simulink model "Hybrid_P2_Parallel_ETE"  (R2017b)
settings: Solver=FixedStepAuto  StartTime=0.0  StopTime=length(Speed)  FixedStep=0.01  MaxStep=0.01  RelTol=1e-3  EnableMultiTasking=on
PostLoadFcn:
  | , if any(exist('dsrtsu_mdlpostloadfcn', 'file') == [2, 3, 6]), try dsrtsu_mdlpostloadfcn('Execute', bdroot); catch fprintf('Error in PostLoadFcn (dsrtsu_mdlpostloadfcn) for model "%s":\n %s\n', bdroot, lasterr); end, end,
undefined symbols (not defined in the file): Actuators, APP1_OOR, APP2_OOR, APP_Mismatch, Brk_Flt, cal, ClutchEngag, CycLength, CycNmb, DiscIntNeverNeededParam, eng, Engine, EngOverTemp, ENGTRQ_MSMCH_Degraded_CP, ENGTRQ_MSMCH_ErrCritical_CP, ENGTRQ_MSMCH_LimpHome_CP, EngTrqMismatch, ess, ESSOverTemp, gb, Gearbox, KeyPos_Flt, lib_Actuators, lib_EMachine_2017a, lib_Sensors_2017a, Loss, LossCAN, Machine, MCUOverTemp, mot, MotDirMismatch, MotOverTemp, MotTrqMismatch, PRNDL_Flt, Ratio, RegenFault, Scope_new, Scopes1, Sensors, Spd, StopIndex, t_amb, time, tloop
libraries: simulink x117, EC2_libraries x9, powerlib_meascontrol x2, CalculationGallon x1, lib_Chassis x1, lib_DCDC x1, lib_Differential x1, lib_HVESS x1, lib_Engine x1, lib_OBC x1, lib_Transmission x1, Transmission_Validation x1
(part 6 of 10)

== system Hybrid_P2_Parallel_ETE/Controller_with_Transmission_Manager1/HSC/Powertrain Manager/Torque Distribution1/Supervisory  Control  Logic1/VehReady.CD_Mode.Brake_mode.MotTrqCalc2 ==
  note: Regenerative braking:
      | Regenerative braking should be allowed under specific chassis speed:
      | chas_spd_below_no_regen= 1.5;
      | chas_spd_above_full_regen = 3;
      | ess_soc_above_regen_forbidden = .92;  % ESS SOC above which regen braking is forbidden
      | ess_soc_above_regen_allowed = .9;% ESS SOC above which regen braking is allowed
  ShftLvrPos : Inport
  TransRatio : Inport  Port=2
  f : TriggerPort  TriggerType=function-call  VariantControl=(inherit)
      settings: CopyFcn=Stateflow.SLINSF.SimulinkMan.removeBlockPreDeleteFcn  PreDeleteFcn=Stateflow.SLINSF.SimulinkMan.unsafePredeleteFcn
  Constant : Constant  Value=0
  Constant1 : Constant  Value=0
  Constant2 : Constant  Value=fd.plant.init.ratio
  Divide2 : Product  Inputs=***
  Idle_torque_Regen : Constant  Value=0
  Index Vector : MultiPortSwitch  DataPortOrder=Zero-based contiguous  Inputs=5  zeroidx=on
  T : Outport
  wires:
  ShftLvrPos/1 -> Index Vector/1
  [TrqCalc] -> Index Vector/4  "R"
  [TrqCalc] -> Index Vector/6  "D"
  Index Vector/1 -> T/1
  Constant/1 -> Index Vector/2  "Between Ranges"
  Constant1/1 -> Index Vector/3  "P"
  [TrqCalc] -> Index Vector/5  "N"
  Constant2/1 -> Divide2/1
  TransRatio/1 -> Divide2/3
  Divide2/1 -> [TrqCalc]  "motor"
  Idle_torque_Regen/1 -> Divide2/2

== system Hybrid_P2_Parallel_ETE/Controller_with_Transmission_Manager1/HSC/Powertrain Manager/Torque Distribution1/Supervisory  Control  Logic1/VehReady.CD_Mode.Drive_mode.MotTrqCalc2 ==
  APP : Inport
  ShftLvrPos : Inport  Port=2
  DrvIntdAxleTrq : Inport  Port=3
  TransRatio : Inport  Port=4
  f : TriggerPort  TriggerType=function-call  VariantControl=(inherit)
      settings: CopyFcn=Stateflow.SLINSF.SimulinkMan.removeBlockPreDeleteFcn  PreDeleteFcn=Stateflow.SLINSF.SimulinkMan.unsafePredeleteFcn
  APPMapLinear : Lookup_n-D  NumberOfTableDimensions=1  BreakpointsForDimension1=[0,1,2,3,4,5,6,7,8,9,10,11,12,13,14,15,16,17,18,19,20,21,22,23,24,25,26,27,28,29,30,31,32,33,34,35,36,37,38,39,40,41,42,43,44,45,46,47,48,49,50,51,52,53,54,55,56,57,58,59,60,70,80,90,100]  Table=[10.5,10.5,10.5,10.5,11,11,11.5,11.5,12,12,12,15,20,25,30,35,40,45,50,55,65,75,85,95,105,115,116,117,118,119,120,121,122,123,124,125,135,140,145,145,150,150,155,160,165,170,175,180,190,195,200,205,210,215,220,225,230,235,240,245,250,275,300,325,350]  ExtrapMethod=Clip  UseLastTableValue=on  InternalRulePriority=Speed  RndMeth=Simplest  InputSameDT=on
  APPMapSelectSW : Constant
  APPOriginal : Lookup_n-D  NumberOfTableDimensions=1  BreakpointsForDimension1=[0,1,2,3,4,5,6,7,8,9,10,11,12,13,14,15,16,17,18,19,20,21,22,23,24,25,26,27,28,29,30,31,32,33,34,35,36,37,38,39,40,41,42,43,44,45,46,47,48,49,50,51,52,53,54,55,56,57,58,59,60,61,62,63,100]  Table=[10,10.5,10.5,10.5,11,11,11.5,12,13,16,20,30,35,40,45,55,60,75,85,95,110,130,150,170,190,210,220.471111355289,231.767041614511,242.413193884843,252.338549994152,261.493375150436,269.849766367567,277.401721265812,284.164727247094,290.17487104503,295.487468649722,300.175215607313,304.325857694294,308.039381966595,311.424728183407,314.596020605783,317.668320170009,320.752897035709,323.952023508727,327.353287338782,331.023425391852,335.001677697353,339.292661870046,343.858767906758,348.612073357775,348,348,348,349,349,349,349,350,350,350,350,350,350,350,350]  ExtrapMethod=Clip  UseLastTableValue=on  InternalRulePriority=Speed  RndMeth=Simplest  InputSameDT=on
  APPScaled60% : Lookup_n-D  NumberOfTableDimensions=1  BreakpointsForDimension1=[0,1,2,3,4,5,6,7,8,9,10,11,12,13,14,15,16,17,18,19,20,21,22,23,24,25,26,27,28,29,30,31,32,33,34,35,36,37,38,39,40,41,42,43,44,45,46,47,48,49,50,51,52,53,54,55,56,57,58,59,60,61,62,63,100]  Table="[10.5000000000000\t10.5000000000000\t10.5000000000000\t10.5000000000000\t11\t11\t11\t11.5000000000000\t11.5000000000000\t11.5000000000000\t12\t18\t21\t24\t27\t33\t36\t45\t51\t57\t66\t78\t90\t102\t114\t126\t132.282666800000\t139.060225000000\t145.447916300000\t151.403130000000\t156.896025100000\t161.909859800000\t166.441032800000\t170.498836300000\t174.104922600000\t177.292481200000\t180.105129400000\t182.595514600000\t184.823629200000\t186.854836900000\t188.757612400000\t190.600992100000\t192.451738200000\t194.371214100000\t196.411972400000\t198.614055200000\t201.001006600000\t203.575597100000\t206.315260700000\t209.167244000000\t208.800000000000\t208.800000000000\t208.800000000000\t209.400000000000\t209.400000000000\t209.400000000000\t209.400000000000\t210\t210\t210\t210\t210\t210\t210\t210]"  ExtrapMethod=Clip  UseLastTableValue=on  InternalRulePriority=Speed  RndMeth=Simplest  InputSameDT=on
  APPScaled80% : Lookup_n-D  NumberOfTableDimensions=1  BreakpointsForDimension1=[0,1,2,3,4,5,6,7,8,9,10,11,12,13,14,15,16,17,18,19,20,21,22,23,24,25,26,27,28,29,30,31,32,33,34,35,36,37,38,39,40,41,42,43,44,45,46,47,48,49,50,51,52,53,54,55,56,57,58,59,60,61,62,63,100]  Table="[10.5000000000000\t10.5000000000000\t10.5000000000000\t10.5000000000000\t11\t11\t11\t11.5000000000000\t11.5000000000000\t11.5000000000000\t12\t24\t28\t32\t36\t44\t48\t60\t68\t76\t88\t104\t120\t136\t152\t168\t176.376889100000\t185.413633300000\t193.930555100000\t201.870840000000\t209.194700100000\t215.879813100000\t221.921377000000\t227.331781800000\t232.139896800000\t236.389974900000\t240.140172500000\t243.460686200000\t246.431505600000\t249.139782500000\t251.676816500000\t254.134656100000\t256.602317600000\t259.161618800000\t261.882629900000\t264.818740300000\t268.001342200000\t271.434129500000\t275.087014300000\t278.889658700000\t278.400000000000\t278.400000000000\t278.400000000000\t279.200000000000\t279.200000000000\t279.200000000000\t279.200000000000\t280\t280\t280\t280\t280\t280\t280\t280]"  ExtrapMethod=Clip  UseLastTableValue=on  InternalRulePriority=Speed  RndMeth=Simplest  InputSameDT=on
  Constant : Constant  Value=0
  Constant1 : Constant  Value=0
  Constant4 : Constant  Value=fd.plant.init.ratio
  Divide2 : Product  Inputs=***
  Index Vector : MultiPortSwitch  DataPortOrder=Zero-based contiguous  Inputs=5  zeroidx=on
  MinMax : MinMax  Inputs=2
  Motor idle torque1 : Subsystem
  Multiport Switch : MultiPortSwitch  Inputs=4
  Saturation : Saturate  UpperLimit=inf  LowerLimit=0
  Saturation2 : Saturate  UpperLimit=100  LowerLimit=0
  Switch : Switch  Criteria=u2 > Threshold  Threshold=3.5
  TransRatio2 : InportShadow  Port=4
  drvAPP2CmbTrq1 : Lookup_n-D  Commented=on  NumberOfTableDimensions=1  BreakpointsForDimension1=[0,1,2,3,4,5,6,7,8,9,10,11,12,13,14,15,16,17,18,19,20,21,22,23,24,25,26,27,28,29,30,31,32,33,34,35,36,37,38,39,40,41,42,43,44,45,46,47,48,49,50,51,52,53,54,55,56,57,58,59,60,61,62,63,64,65,66,67,68,69,70,71,72,73,74,75,76,77,78,79,80,81,82,83,84,85,86,87,88,89,90,91,92,93,94,95,96,97,98,99,100]  Table=[5,15,22,30,37,42,47,51,54,57,59,61.5109301707869,66.8139161912932,73.2458196795481,80.8083280139256,89.4586305380063,99.1171613649123,109.674862556403,120.999967676731,132.944305721263,145.349125419852,158.050439914986,170.883891814679,183.68913862014,196.313758528191,208.616676608453,220.471111355289,231.767041614511,242.413193884843,252.338549994152,261.493375150436,269.849766367567,277.401721265812,284.164727247094,290.17487104503,295.487468649722,300.175215607313,304.325857694294,308.039381966595,311.424728183407,314.596020605783,317.668320170009,320.752897035709,323.952023508727,327.353287338782,331.023425391852,335.001677697353,339.292661870046,343.858767906758,348.612073357775,353.405778873103,358.025164123398,362.178064095715,365.484865763984,367.46802513429,367.541104664833,364.997331060762,364.997331060762,364.997331060762,364.997331060762,364.997331060762,364.997331060762,364.997331060762,364.997331060762,364.997331060762,364.997331060762,364.997331060762,364.997331060762,364.997331060762,364.997331060762,364.997331060762,364.997331060762,364.997331060762,364.997331060762,364.997331060762,364.997331060762,364.997331060762,364.997331060762,364.997331060762,364.997331060762,364.997331060762,364.997331060762,364.997331060762,364.997331060762,364.997331060762,364.997331060762,364.997331060762,364.997331060762,364.997331060762,364.997331060762,364.997331060762,364.997331060762,364.997331060762,364.997331060762,364.997331060762,364.997331060762,364.997331060762,364.997331060762,364.997331060762,364.997331060762,364.997331060762]  ExtrapMethod=Clip  UseLastTableValue=on  InternalRulePriority=Speed  RndMeth=Simplest  InputSameDT=on
  MotTrq : Outport
  wires:
  ShftLvrPos/1 -> Index Vector/1
  [TrqCalc] -> Index Vector/4  "R"
  [TrqCalc] -> Index Vector/6  "D"
  Constant/1 -> Index Vector/2  "Between Ranges"
  Constant1/1 -> Index Vector/5  "N"
  Index Vector/1 -> MotTrq/1
  Constant4/1 -> Divide2/2
  DrvIntdAxleTrq/1 -> Saturation/1  "DrvIntdAxleTrq_CD"
  Divide2/1 -> Switch/1
  Switch/1 -> MinMax/2  "MotAxlTrqAvl_CD"
  TransRatio/1 -> Divide2/1
  Saturation/1 -> MinMax/1
  APPOriginal/1 -> Multiport Switch/5
  Saturation2/1 -> Switch/2
  MinMax/1 -> [TrqCalc]  "MotAxlTrqReq_CD"
  Motor idle torque1/1(Out1) -> Switch/3
  [TrqCalc] -> Index Vector/3  "p"
  TransRatio2/1 -> Motor idle torque1/1(In1)
  Multiport Switch/1 -> Divide2/3  "drvAPP2CmbTrq"
  APPScaled80%/1 -> Multiport Switch/4
  APPScaled60%/1 -> Multiport Switch/3
  APPMapSelectSW/1 -> Multiport Switch/1
  APP/1 -> APPMapLinear/1, APPScaled60%/1, APPScaled80%/1, APPOriginal/1, Saturation2/1
  APPMapLinear/1 -> Multiport Switch/2

== system Hybrid_P2_Parallel_ETE/Controller_with_Transmission_Manager1/HSC/Powertrain Manager/Torque Distribution1/Supervisory  Control  Logic1/VehReady.Eng_Charging_NoReg.EngTrq2EngApp ==
  Trq : Inport
  TransRatio : Inport  Port=2
  f : TriggerPort  TriggerType=function-call  VariantControl=(inherit)
      settings: CopyFcn=Stateflow.SLINSF.SimulinkMan.removeBlockPreDeleteFcn  PreDeleteFcn=Stateflow.SLINSF.SimulinkMan.unsafePredeleteFcn
  Compare To Constant : simulink/Logic and Bit Operations/Compare To Constant  relop===  const=0  OutDataTypeStr=boolean
  Constant1 : Constant  Value=eps
  Constant5 : Constant  Value=fd.plant.init.ratio
  Divide1 : Product  Inputs=*//
  EngTrq2EngAPP : Lookup_n-D  NumberOfTableDimensions=1  BreakpointsForDimension1=[0:1:230]  Table="[-0.950562242591810\t-0.861179388327002\t-0.757792747831397\t-0.640901927898975\t-0.511000095283862\t-0.368573976700328\t-0.214103858822793\t-0.0480635882858183\t0.129079428315885\t0.316864224427463\t0.514836273533913\t0.722547489160089\t0.939556224870697\t1.16542727427030\t1.39973187100331\t1.64204768875400\t1.89195884124648\t2.14905588224475\t2.41293580555262\t2.68320204501379\t2.95946447451180\t3.24133940797003\t3.52844959935174\t3.82042424266002\t4.11689897193784\t4.41751586126800\t4.72192342477317\t5.02977661661586\t5.34073683099846\t5.65447190216317\t5.97065610439209\t6.28897015200715\t6.60910119937013\t6.93074284088268\t7.25359511098630\t7.57736448416234\t7.90176387493200\t8.22651263785634\t8.55133656753627\t8.87596789861257\t9.20014530576584\t9.52361390371657\t9.84612524722509\t10.1674373310916\t10.4873145901561\t10.8055278992985\t11.1218545734385\t11.4360783675358\t11.7479894765898\t12.0573845356398\t12.3640666197649\t12.6678452440843\t12.9685363637566\t13.2659623739808\t13.5599521099953\t13.8503408470787\t14.1369703005491\t14.4196886257647\t14.6983504181235\t14.9728167130634\t15.2429549860620\t15.5086391526369\t15.7697495683456\t16.0261730287853\t16.2778027695931\t16.5245384664460\t16.7662862350608\t17.0029586311942\t17.2344746506427\t17.4607597292427\t17.6817457428705\t17.8973710074422\t18.1075802789137\t18.3123247532808\t18.5115620665792\t18.7052562948843\t18.8933779543117\t19.0759040010164\t19.2528178311935\t19.4241092810781\t19.5897746269448\t19.7498165851084\t19.9042443119232\t20.0530734037837\t20.1963258971241\t20.3340302684184\t20.4662214341804\t20.5929407509641\t20.7142360153630\t20.8301614640105\t20.9407777735800\t21.0461520607847\t21.1463578823776\t21.2414752351516\t21.3315905559394\t21.4167967216136\t21.4971930490867\t21.5728852953111\t21.6439856572787\t21.7106127720217\t21.7728917166119\t21.8309540081611\t21.8849376038208\t21.9349869007824\t21.9812527362772\t22.0238923875764\t22.0630695719909\t22.0989544468717\t22.1317236096093\t22.1615600976344\t22.1886533884173\t22.2131993994684\t22.2354004883376\t22.2554654526151\t22.2736095299306\t22.2900543979538\t22.3050281743942\t22.3187654170013\t22.3315071235641\t22.3435007319120\t22.3550001199137\t22.3662656054781\t22.3775639465539\t22.3891683411296\t22.4013584272335\t22.4144202829338\t22.4286464263386\t22.4443358155959\t22.4617938488934\t22.4813323644587\t22.5032696405595\t22.5279303955028\t22.5556457876361\t22.5867534153463\t22.6215973170604\t22.6605279712450\t22.7039022964069\t22.7520836510924\t22.8054418338880\t22.8643530834197\t22.9292000783536\t23.0003719373956\t23.0782642192915\t23.1632789228268\t23.2558244868269\t23.3563157901571\t23.4651741517227\t23.5828273304686\t23.7097095253797\t23.8462613754808\t23.9929299598362\t24.1501687975506\t24.3184378477682\t24.4982035096730\t24.6899386224892\t24.8941224654804\t25.1112407579505\t25.3417856592430\t25.5862557687413\t25.8451561258686\t26.1189982100880\t26.4082999409026\t26.7135856778550\t27.0353862205281\t27.3742388085443\t27.7306871215661\t28.1052812792955\t28.4985778414748\t28.9111398078859\t29.3435366183506\t29.7963441527305\t30.2701447309271\t30.7655271128819\t31.2830864985759\t31.8234245280303\t32.3871492813060\t32.9748752785038\t33.5872234797643\t34.2248212852680\t34.8883025352352\t35.5783075099261\t36.2954829296408\t37.0404819547192\t37.8139641855409\t38.6165956625258\t39.4490488661331\t40.3120027168621\t41.2061425752523\t42.1321602418824\t43.0907539573713\t44.0826284023780\t45.1084946976008\t46.1690704037782\t47.2650795216887\t48.3972524921501\t49.5663261960208\t50.7730439541983\t52.0181555276205\t53.3024171172650\t54.6265913641491\t55.9914473493301\t57.3977605939052\t58.8463130590113\t60.3378931458253\t61.8732956955639\t63.4533219894835\t65.0787797488808\t66.7504831350916\t68.4692527494924\t70.2359156334991\t72.0513052685674\t73.9162615761929\t75.8316309179113\t77.7982660952979\t79.8170263499681\t81.8887773635766\t84.0143912578187\t86.1947465944290\t88.4307283751822\t90.7232280418928\t93.0731434764153\t95.4813790006436\t97.9488453765121\t100\t100\t100\t100\t100\t100\t100\t100]"  ExtrapMethod=Clip  UseLastTableValue=on  InternalRulePriority=Speed  RndMeth=Simplest  InputSameDT=on
  EngTrq2EngAPP1 : Lookup_n-D  Commented=on  NumberOfTableDimensions=1  BreakpointsForDimension1=[0:1:230]  Table="[-0.950562242591810\t-0.861179388327002\t-0.757792747831397\t-0.640901927898975\t-0.511000095283862\t-0.368573976700328\t-0.214103858822793\t-0.0480635882858183\t0.129079428315885\t0.316864224427463\t0.514836273533913\t0.722547489160089\t0.939556224870697\t1.16542727427030\t1.39973187100331\t1.64204768875400\t1.89195884124648\t2.14905588224475\t2.41293580555262\t2.68320204501379\t2.95946447451180\t3.24133940797003\t3.52844959935174\t3.82042424266002\t4.11689897193784\t4.41751586126800\t4.72192342477317\t5.02977661661586\t5.34073683099846\t5.65447190216317\t5.97065610439209\t6.28897015200715\t6.60910119937013\t6.93074284088268\t7.25359511098630\t7.57736448416234\t7.90176387493200\t8.22651263785634\t8.55133656753627\t8.87596789861257\t9.20014530576584\t9.52361390371657\t9.84612524722509\t10.1674373310916\t10.4873145901561\t10.8055278992985\t11.1218545734385\t11.4360783675358\t11.7479894765898\t12.0573845356398\t12.3640666197649\t12.6678452440843\t12.9685363637566\t13.2659623739808\t13.5599521099953\t13.8503408470787\t14.1369703005491\t14.4196886257647\t14.6983504181235\t14.9728167130634\t15.2429549860620\t15.5086391526369\t15.7697495683456\t16.0261730287853\t16.2778027695931\t16.5245384664460\t16.7662862350608\t17.0029586311942\t17.2344746506427\t17.4607597292427\t17.6817457428705\t17.8973710074422\t18.1075802789137\t18.3123247532808\t18.5115620665792\t18.7052562948843\t18.8933779543117\t19.0759040010164\t19.2528178311935\t19.4241092810781\t19.5897746269448\t19.7498165851084\t19.9042443119232\t20.0530734037837\t20.1963258971241\t20.3340302684184\t20.4662214341804\t20.5929407509641\t20.7142360153630\t20.8301614640105\t20.9407777735800\t21.0461520607847\t21.1463578823776\t21.2414752351516\t21.3315905559394\t21.4167967216136\t21.4971930490867\t21.5728852953111\t21.6439856572787\t21.7106127720217\t21.7728917166119\t21.8309540081611\t21.8849376038208\t21.9349869007824\t21.9812527362772\t22.0238923875764\t22.0630695719909\t22.0989544468717\t22.1317236096093\t22.1615600976344\t22.1886533884173\t22.2131993994684\t22.2354004883376\t22.2554654526151\t22.2736095299306\t22.2900543979538\t22.3050281743942\t22.3187654170013\t22.3315071235641\t22.3435007319120\t22.3550001199137\t22.3662656054781\t22.3775639465539\t22.3891683411296\t22.4013584272335\t22.4144202829338\t22.4286464263386\t22.4443358155959\t22.4617938488934\t22.4813323644587\t22.5032696405595\t22.5279303955028\t22.5556457876361\t22.5867534153463\t22.6215973170604\t22.6605279712450\t22.7039022964069\t22.7520836510924\t22.8054418338880\t22.8643530834197\t22.9292000783536\t23.0003719373956\t23.0782642192915\t23.1632789228268\t23.2558244868269\t23.3563157901571\t23.4651741517227\t23.5828273304686\t23.7097095253797\t23.8462613754808\t23.9929299598362\t24.1501687975506\t24.3184378477682\t24.4982035096730\t24.6899386224892\t24.8941224654804\t25.1112407579505\t25.3417856592430\t25.5862557687413\t25.8451561258686\t26.1189982100880\t26.4082999409026\t26.7135856778550\t27.0353862205281\t27.3742388085443\t27.7306871215661\t28.1052812792955\t28.4985778414748\t28.9111398078859\t29.3435366183506\t29.7963441527305\t30.2701447309271\t30.7655271128819\t31.2830864985759\t31.8234245280303\t32.3871492813060\t32.9748752785038\t33.5872234797643\t34.2248212852680\t34.8883025352352\t35.5783075099261\t36.2954829296408\t37.0404819547192\t37.8139641855409\t38.6165956625258\t39.4490488661331\t40.3120027168621\t41.2061425752523\t42.1321602418824\t43.0907539573713\t44.0826284023780\t45.1084946976008\t46.1690704037782\t47.2650795216887\t48.3972524921501\t49.5663261960208\t50.7730439541983\t52.0181555276205\t53.3024171172650\t54.6265913641491\t55.9914473493301\t57.3977605939052\t58.8463130590113\t60.3378931458253\t61.8732956955639\t63.4533219894835\t65.0787797488808\t66.7504831350916\t68.4692527494924\t70.2359156334991\t72.0513052685674\t73.9162615761929\t75.8316309179113\t77.7982660952979\t79.8170263499681\t81.8887773635766\t84.0143912578187\t86.1947465944290\t88.4307283751822\t90.7232280418928\t93.0731434764153\t95.4813790006436\t97.9488453765121\t100\t100\t100\t100\t100\t100\t100\t100]"  ExtrapMethod=Clip  UseLastTableValue=on  InternalRulePriority=Speed  RndMeth=Simplest  InputSameDT=on
  Saturation : Saturate  UpperLimit=100  LowerLimit=0
  Switch : Switch  Criteria=u2 > Threshold
  APP : Outport
  wires:
  Trq/1 -> Divide1/1
  Constant5/1 -> Divide1/2
  Compare To Constant/1 -> Switch/2
  Constant1/1 -> Switch/1
  Switch/1 -> Divide1/3
  Divide1/1 -> EngTrq2EngAPP/1
  TransRatio/1 -> Switch/3, Compare To Constant/1
  EngTrq2EngAPP/1 -> Saturation/1
  Saturation/1 -> APP/1

== system Hybrid_P2_Parallel_ETE/Controller_with_Transmission_Manager1/HSC/Powertrain Manager/Torque Distribution1/Supervisory  Control  Logic1/VehReady.Eng_Charging_NoReg.EngTrqCalc ==
  EngSpeed : Inport
  APP : Inport  Port=2
  ShftLvrPos : Inport  Port=3
  DrvIntdAxleTrq : Inport  Port=4
  TransRatio : Inport  Port=5
  f : TriggerPort  TriggerType=function-call  VariantControl=(inherit)
      settings: CopyFcn=Stateflow.SLINSF.SimulinkMan.removeBlockPreDeleteFcn  PreDeleteFcn=Stateflow.SLINSF.SimulinkMan.unsafePredeleteFcn
  APP Derating : Lookup_n-D  NumberOfTableDimensions=1  BreakpointsForDimension1=[0 1 2 3 5 7]  Table=[0 0.1 0.3 0.5 0.7 1]  ExtrapMethod=Clip  UseLastTableValue=on  InternalRulePriority=Speed  RndMeth=Simplest  InputSameDT=on
  Constant : Constant  Value=0
  Constant2 : Constant  Value=0
  Constant3 : Constant  Value=fd.plant.init.ratio
  Divide : Product  Inputs=**
  Divide2 : Product  Inputs=***
  Engine Max Trq : Lookup_n-D  NumberOfTableDimensions=1  BreakpointsForDimension1="[600\t800\t1000\t1200\t1400\t1600\t1800\t2000\t2200\t2400\t2600\t2800\t3000\t3200\t3400\t3600\t3800\t4000\t4250\t4500\t4750\t5000\t5250\t5500\t5750\t6000\t6250\t6500]"  Table="[83.7900000000000\t136.760000000000\t140\t152.010000000000\t171.590000000000\t185.900000000000\t198.400000000000\t197.360000000000\t200.550000000000\t202.260000000000\t215.080000000000\t204.810000000000\t204.520000000000\t208.100000000000\t211.520000000000\t210.560000000000\t214.100000000000\t213.470000000000\t208.730000000000\t208.430000000000\t208.670000000000\t231.210000000000\t228.310000000000\t225.330000000000\t220.520000000000\t211.210000000000\t204.190000000000\t151.770000000000]"  ExtrapMethod=Clip  UseLastTableValue=on  InternalRulePriority=Speed  RndMeth=Simplest  InputSameDT=on
  MinMax : MinMax  Function=max  Inputs=2
  Shifter : MultiPortSwitch  DataPortOrder=Zero-based contiguous  Inputs=5  zeroidx=on
  Trq : Outport
  wires:
  EngSpeed/1 -> Engine Max Trq/1
  APP/1 -> APP Derating/1
  APP Derating/1 -> Divide/2
  ShftLvrPos/1 -> Shifter/1
  [TrqCalc] -> Shifter/4  "R"
  [TrqCalc] -> Shifter/6  "D"
  Constant/1 -> Shifter/2  "Between Ranges"
  [TrqCalc] -> Shifter/3  "P"
  Constant2/1 -> Shifter/5  "N"
  Shifter/1 -> Trq/1
  Constant3/1 -> Divide2/1
  Divide/1 -> Divide2/2
  Divide2/1 -> MinMax/2  "engine"
  TransRatio/1 -> Divide2/3
  DrvIntdAxleTrq/1 -> MinMax/1  "driver"
  MinMax/1 -> [TrqCalc]
  Engine Max Trq/1 -> Divide/1

== system Hybrid_P2_Parallel_ETE/Controller_with_Transmission_Manager1/HSC/Powertrain Manager/Torque Distribution1/Supervisory  Control  Logic1/VehReady.Eng_Charging_NoReg.MotTrqCalc ==
  ShftLvrPos : Inport
  DrvIntdAxleTrq : Inport  Port=2
  Trq : Inport  Port=3
  SoC : Inport  Port=4
  Volt : Inport  Port=5
  f : TriggerPort  TriggerType=function-call  VariantControl=(inherit)
      settings: CopyFcn=Stateflow.SLINSF.SimulinkMan.removeBlockPreDeleteFcn  PreDeleteFcn=Stateflow.SLINSF.SimulinkMan.unsafePredeleteFcn
  Add : Sum  Inputs=-+
  Compare To Constant : simulink/Logic and Bit Operations/Compare To Constant  relop=>=  const=80  OutDataTypeStr=boolean
  Compare To Constant1 : simulink/Logic and Bit Operations/Compare To Constant  relop=>=  const=415  OutDataTypeStr=boolean
  Constant : Constant  Value=0
  Constant2 : Constant  Value=0
  Logical Operator : Logic  Operator=OR  AllPortsSameDT=off  OutDataTypeStr=boolean
  NoMotTr	q : Constant  Value=0
  Shifter : MultiPortSwitch  DataPortOrder=Zero-based contiguous  Inputs=5  zeroidx=on
  Switch : Switch  Criteria=u2 > Threshold
  MotTrq : Outport
  wires:
  ShftLvrPos/1 -> Shifter/1
  [TrqCalc] -> Shifter/4  "R"
  [TrqCalc] -> Shifter/6  "D"
  Constant/1 -> Shifter/2  "Between Ranges"
  [TrqCalc] -> Shifter/3  "P"
  Constant2/1 -> Shifter/5  "N"
  Shifter/1 -> MotTrq/1
  DrvIntdAxleTrq/1 -> Add/2
  Trq/1 -> Add/1
  SoC/1 -> Compare To Constant/1
  Compare To Constant/1 -> Logical Operator/1
  Logical Operator/1 -> Switch/2
  Switch/1 -> [TrqCalc]
  Add/1 -> Switch/3
  NoMotTr	q/1 -> Switch/1
  Volt/1 -> Compare To Constant1/1
  Compare To Constant1/1 -> Logical Operator/2

== system Hybrid_P2_Parallel_ETE/Controller_with_Transmission_Manager1/HSC/Powertrain Manager/Torque Distribution1/Supervisory  Control  Logic1/VehReady.Eng_Charging_Stat.EngTrq2EngApp ==
  Trq : Inport
  TransRatio : Inport  Port=2
  f : TriggerPort  TriggerType=function-call  VariantControl=(inherit)
      settings: CopyFcn=Stateflow.SLINSF.SimulinkMan.removeBlockPreDeleteFcn  PreDeleteFcn=Stateflow.SLINSF.SimulinkMan.unsafePredeleteFcn
  Compare To Constant : simulink/Logic and Bit Operations/Compare To Constant  relop===  const=0  OutDataTypeStr=boolean
  Constant1 : Constant  Value=eps
  Constant5 : Constant  Value=fd.plant.init.ratio
  Divide1 : Product  Inputs=*//
  EngTrq2EngAPP : Lookup_n-D  NumberOfTableDimensions=1  BreakpointsForDimension1=[0:1:230]  Table="[-0.950562242591810\t-0.861179388327002\t-0.757792747831397\t-0.640901927898975\t-0.511000095283862\t-0.368573976700328\t-0.214103858822793\t-0.0480635882858183\t0.129079428315885\t0.316864224427463\t0.514836273533913\t0.722547489160089\t0.939556224870697\t1.16542727427030\t1.39973187100331\t1.64204768875400\t1.89195884124648\t2.14905588224475\t2.41293580555262\t2.68320204501379\t2.95946447451180\t3.24133940797003\t3.52844959935174\t3.82042424266002\t4.11689897193784\t4.41751586126800\t4.72192342477317\t5.02977661661586\t5.34073683099846\t5.65447190216317\t5.97065610439209\t6.28897015200715\t6.60910119937013\t6.93074284088268\t7.25359511098630\t7.57736448416234\t7.90176387493200\t8.22651263785634\t8.55133656753627\t8.87596789861257\t9.20014530576584\t9.52361390371657\t9.84612524722509\t10.1674373310916\t10.4873145901561\t10.8055278992985\t11.1218545734385\t11.4360783675358\t11.7479894765898\t12.0573845356398\t12.3640666197649\t12.6678452440843\t12.9685363637566\t13.2659623739808\t13.5599521099953\t13.8503408470787\t14.1369703005491\t14.4196886257647\t14.6983504181235\t14.9728167130634\t15.2429549860620\t15.5086391526369\t15.7697495683456\t16.0261730287853\t16.2778027695931\t16.5245384664460\t16.7662862350608\t17.0029586311942\t17.2344746506427\t17.4607597292427\t17.6817457428705\t17.8973710074422\t18.1075802789137\t18.3123247532808\t18.5115620665792\t18.7052562948843\t18.8933779543117\t19.0759040010164\t19.2528178311935\t19.4241092810781\t19.5897746269448\t19.7498165851084\t19.9042443119232\t20.0530734037837\t20.1963258971241\t20.3340302684184\t20.4662214341804\t20.5929407509641\t20.7142360153630\t20.8301614640105\t20.9407777735800\t21.0461520607847\t21.1463578823776\t21.2414752351516\t21.3315905559394\t21.4167967216136\t21.4971930490867\t21.5728852953111\t21.6439856572787\t21.7106127720217\t21.7728917166119\t21.8309540081611\t21.8849376038208\t21.9349869007824\t21.9812527362772\t22.0238923875764\t22.0630695719909\t22.0989544468717\t22.1317236096093\t22.1615600976344\t22.1886533884173\t22.2131993994684\t22.2354004883376\t22.2554654526151\t22.2736095299306\t22.2900543979538\t22.3050281743942\t22.3187654170013\t22.3315071235641\t22.3435007319120\t22.3550001199137\t22.3662656054781\t22.3775639465539\t22.3891683411296\t22.4013584272335\t22.4144202829338\t22.4286464263386\t22.4443358155959\t22.4617938488934\t22.4813323644587\t22.5032696405595\t22.5279303955028\t22.5556457876361\t22.5867534153463\t22.6215973170604\t22.6605279712450\t22.7039022964069\t22.7520836510924\t22.8054418338880\t22.8643530834197\t22.9292000783536\t23.0003719373956\t23.0782642192915\t23.1632789228268\t23.2558244868269\t23.3563157901571\t23.4651741517227\t23.5828273304686\t23.7097095253797\t23.8462613754808\t23.9929299598362\t24.1501687975506\t24.3184378477682\t24.4982035096730\t24.6899386224892\t24.8941224654804\t25.1112407579505\t25.3417856592430\t25.5862557687413\t25.8451561258686\t26.1189982100880\t26.4082999409026\t26.7135856778550\t27.0353862205281\t27.3742388085443\t27.7306871215661\t28.1052812792955\t28.4985778414748\t28.9111398078859\t29.3435366183506\t29.7963441527305\t30.2701447309271\t30.7655271128819\t31.2830864985759\t31.8234245280303\t32.3871492813060\t32.9748752785038\t33.5872234797643\t34.2248212852680\t34.8883025352352\t35.5783075099261\t36.2954829296408\t37.0404819547192\t37.8139641855409\t38.6165956625258\t39.4490488661331\t40.3120027168621\t41.2061425752523\t42.1321602418824\t43.0907539573713\t44.0826284023780\t45.1084946976008\t46.1690704037782\t47.2650795216887\t48.3972524921501\t49.5663261960208\t50.7730439541983\t52.0181555276205\t53.3024171172650\t54.6265913641491\t55.9914473493301\t57.3977605939052\t58.8463130590113\t60.3378931458253\t61.8732956955639\t63.4533219894835\t65.0787797488808\t66.7504831350916\t68.4692527494924\t70.2359156334991\t72.0513052685674\t73.9162615761929\t75.8316309179113\t77.7982660952979\t79.8170263499681\t81.8887773635766\t84.0143912578187\t86.1947465944290\t88.4307283751822\t90.7232280418928\t93.0731434764153\t95.4813790006436\t97.9488453765121\t100\t100\t100\t100\t100\t100\t100\t100]"  ExtrapMethod=Clip  UseLastTableValue=on  InternalRulePriority=Speed  RndMeth=Simplest  InputSameDT=on
  EngTrq2EngAPP1 : Lookup_n-D  Commented=on  NumberOfTableDimensions=1  BreakpointsForDimension1=[0:1:230]  Table="[-0.950562242591810\t-0.861179388327002\t-0.757792747831397\t-0.640901927898975\t-0.511000095283862\t-0.368573976700328\t-0.214103858822793\t-0.0480635882858183\t0.129079428315885\t0.316864224427463\t0.514836273533913\t0.722547489160089\t0.939556224870697\t1.16542727427030\t1.39973187100331\t1.64204768875400\t1.89195884124648\t2.14905588224475\t2.41293580555262\t2.68320204501379\t2.95946447451180\t3.24133940797003\t3.52844959935174\t3.82042424266002\t4.11689897193784\t4.41751586126800\t4.72192342477317\t5.02977661661586\t5.34073683099846\t5.65447190216317\t5.97065610439209\t6.28897015200715\t6.60910119937013\t6.93074284088268\t7.25359511098630\t7.57736448416234\t7.90176387493200\t8.22651263785634\t8.55133656753627\t8.87596789861257\t9.20014530576584\t9.52361390371657\t9.84612524722509\t10.1674373310916\t10.4873145901561\t10.8055278992985\t11.1218545734385\t11.4360783675358\t11.7479894765898\t12.0573845356398\t12.3640666197649\t12.6678452440843\t12.9685363637566\t13.2659623739808\t13.5599521099953\t13.8503408470787\t14.1369703005491\t14.4196886257647\t14.6983504181235\t14.9728167130634\t15.2429549860620\t15.5086391526369\t15.7697495683456\t16.0261730287853\t16.2778027695931\t16.5245384664460\t16.7662862350608\t17.0029586311942\t17.2344746506427\t17.4607597292427\t17.6817457428705\t17.8973710074422\t18.1075802789137\t18.3123247532808\t18.5115620665792\t18.7052562948843\t18.8933779543117\t19.0759040010164\t19.2528178311935\t19.4241092810781\t19.5897746269448\t19.7498165851084\t19.9042443119232\t20.0530734037837\t20.1963258971241\t20.3340302684184\t20.4662214341804\t20.5929407509641\t20.7142360153630\t20.8301614640105\t20.9407777735800\t21.0461520607847\t21.1463578823776\t21.2414752351516\t21.3315905559394\t21.4167967216136\t21.4971930490867\t21.5728852953111\t21.6439856572787\t21.7106127720217\t21.7728917166119\t21.8309540081611\t21.8849376038208\t21.9349869007824\t21.9812527362772\t22.0238923875764\t22.0630695719909\t22.0989544468717\t22.1317236096093\t22.1615600976344\t22.1886533884173\t22.2131993994684\t22.2354004883376\t22.2554654526151\t22.2736095299306\t22.2900543979538\t22.3050281743942\t22.3187654170013\t22.3315071235641\t22.3435007319120\t22.3550001199137\t22.3662656054781\t22.3775639465539\t22.3891683411296\t22.4013584272335\t22.4144202829338\t22.4286464263386\t22.4443358155959\t22.4617938488934\t22.4813323644587\t22.5032696405595\t22.5279303955028\t22.5556457876361\t22.5867534153463\t22.6215973170604\t22.6605279712450\t22.7039022964069\t22.7520836510924\t22.8054418338880\t22.8643530834197\t22.9292000783536\t23.0003719373956\t23.0782642192915\t23.1632789228268\t23.2558244868269\t23.3563157901571\t23.4651741517227\t23.5828273304686\t23.7097095253797\t23.8462613754808\t23.9929299598362\t24.1501687975506\t24.3184378477682\t24.4982035096730\t24.6899386224892\t24.8941224654804\t25.1112407579505\t25.3417856592430\t25.5862557687413\t25.8451561258686\t26.1189982100880\t26.4082999409026\t26.7135856778550\t27.0353862205281\t27.3742388085443\t27.7306871215661\t28.1052812792955\t28.4985778414748\t28.9111398078859\t29.3435366183506\t29.7963441527305\t30.2701447309271\t30.7655271128819\t31.2830864985759\t31.8234245280303\t32.3871492813060\t32.9748752785038\t33.5872234797643\t34.2248212852680\t34.8883025352352\t35.5783075099261\t36.2954829296408\t37.0404819547192\t37.8139641855409\t38.6165956625258\t39.4490488661331\t40.3120027168621\t41.2061425752523\t42.1321602418824\t43.0907539573713\t44.0826284023780\t45.1084946976008\t46.1690704037782\t47.2650795216887\t48.3972524921501\t49.5663261960208\t50.7730439541983\t52.0181555276205\t53.3024171172650\t54.6265913641491\t55.9914473493301\t57.3977605939052\t58.8463130590113\t60.3378931458253\t61.8732956955639\t63.4533219894835\t65.0787797488808\t66.7504831350916\t68.4692527494924\t70.2359156334991\t72.0513052685674\t73.9162615761929\t75.8316309179113\t77.7982660952979\t79.8170263499681\t81.8887773635766\t84.0143912578187\t86.1947465944290\t88.4307283751822\t90.7232280418928\t93.0731434764153\t95.4813790006436\t97.9488453765121\t100\t100\t100\t100\t100\t100\t100\t100]"  ExtrapMethod=Clip  UseLastTableValue=on  InternalRulePriority=Speed  RndMeth=Simplest  InputSameDT=on
  Saturation : Saturate  UpperLimit=100  LowerLimit=0
  Switch : Switch  Criteria=u2 > Threshold
  APP : Outport
  wires:
  Trq/1 -> Divide1/1
  Constant5/1 -> Divide1/2
  Compare To Constant/1 -> Switch/2
  Constant1/1 -> Switch/1
  Switch/1 -> Divide1/3
  Divide1/1 -> EngTrq2EngAPP/1
  TransRatio/1 -> Switch/3, Compare To Constant/1
  EngTrq2EngAPP/1 -> Saturation/1
  Saturation/1 -> APP/1

== system Hybrid_P2_Parallel_ETE/Controller_with_Transmission_Manager1/HSC/Powertrain Manager/Torque Distribution1/Supervisory  Control  Logic1/VehReady.Eng_Charging_Stat.EngTrqCalc ==
  EngSpeed : Inport
  ShftLvrPos : Inport  Port=2
  DrvIntdAxleTrq : Inport  Port=3
  TransRatio : Inport  Port=4
  f : TriggerPort  TriggerType=function-call  VariantControl=(inherit)
      settings: CopyFcn=Stateflow.SLINSF.SimulinkMan.removeBlockPreDeleteFcn  PreDeleteFcn=Stateflow.SLINSF.SimulinkMan.unsafePredeleteFcn
  Constant{,1..2,4} (4 alike) : Constant  Value=0
  Constant3 : Constant  Value=fd.plant.init.ratio
  Divide2 : Product  Inputs=***
  Engine Max Trq : Lookup_n-D  NumberOfTableDimensions=1  BreakpointsForDimension1="[600\t800\t1000\t1200\t1400\t1600\t1800\t2000\t2200\t2400\t2600\t2800\t3000\t3200\t3400\t3600\t3800\t4000\t4250\t4500\t4750\t5000\t5250\t5500\t5750\t6000\t6250\t6500]"  Table="[83.7900000000000\t136.760000000000\t140\t152.010000000000\t171.590000000000\t185.900000000000\t198.400000000000\t197.360000000000\t200.550000000000\t202.260000000000\t215.080000000000\t204.810000000000\t204.520000000000\t208.100000000000\t211.520000000000\t210.560000000000\t214.100000000000\t213.470000000000\t208.730000000000\t208.430000000000\t208.670000000000\t231.210000000000\t228.310000000000\t225.330000000000\t220.520000000000\t211.210000000000\t204.190000000000\t151.770000000000]"  ExtrapMethod=Clip  UseLastTableValue=on  InternalRulePriority=Speed  RndMeth=Simplest  InputSameDT=on
  MinMax : MinMax  Function=max  Inputs=2
  Multiply by Zero fix : Subsystem
  Shifter : MultiPortSwitch  DataPortOrder=Zero-based contiguous  Inputs=5  zeroidx=on
  Trq : Outport
  wires:
  EngSpeed/1 -> Engine Max Trq/1
  ShftLvrPos/1 -> Shifter/1
  Constant1/1 -> Shifter/4  "R"
  Constant4/1 -> Shifter/6  "D"
  Constant/1 -> Shifter/2  "Between Ranges"
  [TrqCalc] -> Shifter/3  "P"
  Constant2/1 -> Shifter/5  "N"
  Shifter/1 -> Trq/1
  Constant3/1 -> Divide2/1
  Engine Max Trq/1 -> Divide2/2  "EngMaxTrq_Map"
  Divide2/1 -> MinMax/2  "engine"
  TransRatio/1 -> Multiply by Zero fix/1(In1)
  DrvIntdAxleTrq/1 -> MinMax/1  "driver"
  MinMax/1 -> [TrqCalc]  "EngActAxlTrq"
  Multiply by Zero fix/1(Out1) -> Divide2/3

== system Hybrid_P2_Parallel_ETE/Controller_with_Transmission_Manager1/HSC/Powertrain Manager/Torque Distribution1/Supervisory  Control  Logic1/VehReady.Eng_Charging_Stat.MotTrqCalc ==
  ShftLvrPos : Inport
  DrvIntdAxleTrq : Inport  Port=2
  Trq : Inport  Port=3
  SoC : Inport  Port=4
  Volt : Inport  Port=5
  APP : Inport  Port=6
  f : TriggerPort  TriggerType=function-call  VariantControl=(inherit)
      settings: CopyFcn=Stateflow.SLINSF.SimulinkMan.removeBlockPreDeleteFcn  PreDeleteFcn=Stateflow.SLINSF.SimulinkMan.unsafePredeleteFcn
  Add : Sum  Inputs=-+
  Compare To Constant : simulink/Logic and Bit Operations/Compare To Constant  relop=>=  const=80  OutDataTypeStr=boolean
  Compare To Constant1 : simulink/Logic and Bit Operations/Compare To Constant  relop=>=  const=415  OutDataTypeStr=boolean
  Compare To Constant2 : simulink/Logic and Bit Operations/Compare To Constant  relop=<  const=3  OutDataTypeStr=boolean
  Constant{,1..3} (4 alike) : Constant  Value=0
  Logical Operator : Logic  Operator=OR  AllPortsSameDT=off  OutDataTypeStr=boolean
  MaxChargeTrq : Constant  Value=-45
  MinChargeTrq : Constant  Value=0
  NoMotTr	q : Constant  Value=0
  Saturation Dynamic : simulink/Discontinuities/Saturation Dynamic  OutMin=[]  OutMax=[]  OutDataTypeStr=Inherit: Same as second input  OutDataType=fixdt(1, 16)  OutScaling=2^-10  DoSatur=off
  Shifter : MultiPortSwitch  DataPortOrder=Zero-based contiguous  Inputs=5  zeroidx=on
  Switch : Switch  Criteria=u2 > Threshold
  Switch1 : Switch  Criteria=u2 > Threshold
  MotTrq : Outport
  wires:
  ShftLvrPos/1 -> Shifter/1
  Constant1/1 -> Shifter/4  "R"
  Constant3/1 -> Shifter/6  "D"
  Constant/1 -> Shifter/2  "Between Ranges"
  [TrqCalc] -> Shifter/3  "P"
  Constant2/1 -> Shifter/5  "N"
  Shifter/1 -> MotTrq/1
  DrvIntdAxleTrq/1 -> Add/2
  Trq/1 -> Add/1
  SoC/1 -> Compare To Constant/1
  Compare To Constant/1 -> Logical Operator/1
  Logical Operator/1 -> Switch/2
  Add/1 -> Switch/3
  NoMotTr	q/1 -> Switch/1
  Volt/1 -> Compare To Constant1/1
  Compare To Constant1/1 -> Logical Operator/2
  APP/1 -> Compare To Constant2/1
  Compare To Constant2/1 -> Switch1/2
  Switch1/1 -> [TrqCalc]  "MotAxlTrq_ChargingAfterSaturation"
  Saturation Dynamic/1 -> Switch1/1
  MinChargeTrq/1 -> Saturation Dynamic/1
  Switch/1 -> Switch1/3, Saturation Dynamic/2  "MotAxlTrq_ChargingBeforeSaturation"
  MaxChargeTrq/1 -> Saturation Dynamic/3

== system Hybrid_P2_Parallel_ETE/Controller_with_Transmission_Manager1/HSC/Powertrain Manager/Torque Distribution1/Supervisory  Control  Logic1/VehReady.Engine_Charge.Brake_mode1.MotTrqCalc1 ==
  note: Regenerative braking:
      | Regenerative braking should be allowed under specific chassis speed:
      | chas_spd_below_no_regen= 1.5;
      | chas_spd_above_full_regen = 3;
      | ess_soc_above_regen_forbidden = .92;  % ESS SOC above which regen braking is forbidden
      | ess_soc_above_regen_allowed = .9;% ESS SOC above which regen braking is allowed
  BPP : Inport
  VehSpd : Inport  Port=2
  ShftLvrPos : Inport  Port=3
  MotSpeed : Inport  Port=4
  TransRatio : Inport  Port=5
  IntdAxleTrq : Inport  Port=6
  f : TriggerPort  TriggerType=function-call  VariantControl=(inherit)
      settings: CopyFcn=Stateflow.SLINSF.SimulinkMan.removeBlockPreDeleteFcn  PreDeleteFcn=Stateflow.SLINSF.SimulinkMan.unsafePredeleteFcn
  "% to 1 " : Gain  Gain=1/100
  Constant : Constant  Value=0
  Constant1 : Constant  Value=0
  Constant2 : Constant  Value=fd.plant.init.ratio
  Divide : Product  Inputs=***
  Divide2 : Product  Inputs=***
  Index Vector : MultiPortSwitch  DataPortOrder=Zero-based contiguous  Inputs=5  zeroidx=on
  MinMax : MinMax  Function=max  Inputs=2
  Peak trq max - Regen : Lookup  InputValues=mot.plant.init.regen.trq_max.idx1_spd  Table=mot.plant.init.regen.trq_max.map  LookUpMeth=Interpolation-Use End Values  SaturateOnIntegerOverflow=on
  Regen Trq Derating : Lookup_n-D  Commented=on  NumberOfTableDimensions=1  BreakpointsForDimension1=[0 20 30 40 50]  Table=[0 0.025 0.05 0.1 1]  ExtrapMethod=Clip  UseLastTableValue=on  InternalRulePriority=Speed  RndMeth=Simplest  InputSameDT=on
  Regen Trq Derating1 : Lookup_n-D  NumberOfTableDimensions=1  BreakpointsForDimension1=[0 10 11 200]  Table=[0 0.5 1 1]  ExtrapMethod=Clip  UseLastTableValue=on  InternalRulePriority=Speed  RndMeth=Simplest  InputSameDT=on
  Regen_derat_overri : Constant  Value=0
  Regen_derat_value : Constant  Value=0.5
  Switch : Switch  Criteria=u2 > Threshold
  limit to 100Nm : Saturate  UpperLimit=0  LowerLimit=-100
  T : Outport
  wires:
  BPP/1 -> "% to 1 "/1
  "% to 1 "/1 -> Divide/1
  Divide/1 -> limit to 100Nm/1
  VehSpd/1 -> Regen Trq Derating1/1
  ShftLvrPos/1 -> Index Vector/1
  [TrqCalc] -> Index Vector/4  "R"
  [TrqCalc] -> Index Vector/6  "D"
  Index Vector/1 -> T/1
  Constant/1 -> Index Vector/2  "Between Ranges"
  Constant1/1 -> Index Vector/3  "P"
  [TrqCalc] -> Index Vector/5  "N"
  MotSpeed/1 -> Peak trq max - Regen/1  "RPM"
  Peak trq max - Regen/1 -> Divide/2
  Constant2/1 -> Divide2/1
  limit to 100Nm/1 -> Divide2/2
  TransRatio/1 -> Divide2/3
  Divide2/1 -> MinMax/2  "motor"
  Regen Trq Derating1/1 -> Switch/3
  Regen_derat_overri/1 -> Switch/2
  Switch/1 -> Divide/3
  Regen_derat_value/1 -> Switch/1
  IntdAxleTrq/1 -> MinMax/1
  MinMax/1 -> [TrqCalc]

== system Hybrid_P2_Parallel_ETE/Controller_with_Transmission_Manager1/HSC/Powertrain Manager/Torque Distribution1/Supervisory  Control  Logic1/VehReady.Engine_Charge.Brake_mode1.MotTrqCalc2 ==
  note: Regenerative braking:
      | Regenerative braking should be allowed under specific chassis speed:
      | chas_spd_below_no_regen= 1.5;
      | chas_spd_above_full_regen = 3;
      | ess_soc_above_regen_forbidden = .92;  % ESS SOC above which regen braking is forbidden
      | ess_soc_above_regen_allowed = .9;% ESS SOC above which regen braking is allowed
  ShftLvrPos : Inport
  TransRatio : Inport  Port=2
  f : TriggerPort  TriggerType=function-call  VariantControl=(inherit)
      settings: CopyFcn=Stateflow.SLINSF.SimulinkMan.removeBlockPreDeleteFcn  PreDeleteFcn=Stateflow.SLINSF.SimulinkMan.unsafePredeleteFcn
  Constant : Constant  Value=0
  Constant1 : Constant  Value=0
  Constant2 : Constant  Value=fd.plant.init.ratio
  Divide2 : Product  Inputs=***
  Idle_torque_Regen : Constant  Value=0
  Index Vector : MultiPortSwitch  DataPortOrder=Zero-based contiguous  Inputs=5  zeroidx=on
  T : Outport
  wires:
  ShftLvrPos/1 -> Index Vector/1
  [TrqCalc] -> Index Vector/4  "R"
  [TrqCalc] -> Index Vector/6  "D"
  Index Vector/1 -> T/1
  Constant/1 -> Index Vector/2  "Between Ranges"
  Constant1/1 -> Index Vector/3  "P"
  [TrqCalc] -> Index Vector/5  "N"
  Constant2/1 -> Divide2/1
  TransRatio/1 -> Divide2/3
  Divide2/1 -> [TrqCalc]  "motor"
  Idle_torque_Regen/1 -> Divide2/2
